simulink model "escooter_behavior_diagram"  (R2025b)
settings: Solver=VariableStepDiscrete  StartTime=0.0  StopTime=10.0  MaxStep=Inf  RelTol=1e-3
settings Model: Creator=320236370  LastModifiedBy=320236370

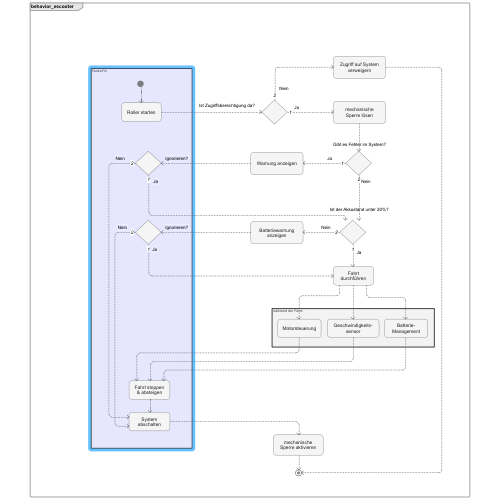
[thumbnail: Simulink's stored preview of the top-level diagram]
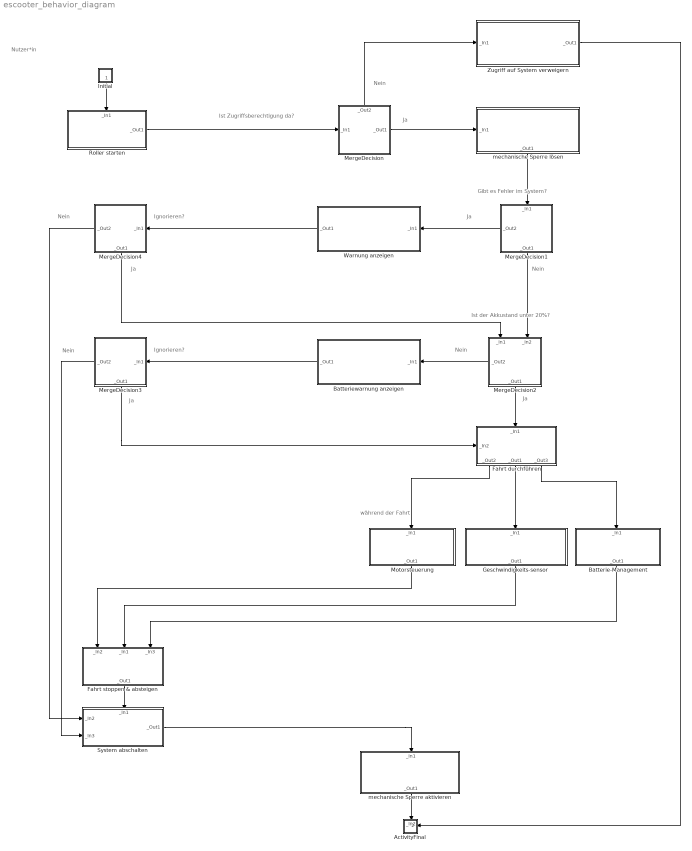
== system escooter_behavior_diagram ==
  note: Nein
  note: Nein
  note: Nein
  note: Ja
  note: Ignorieren?
  note: Ja
  note: Nutzer*in
  note: Nein
  note: Ja
  note: Ja
  note: während der Fahrt
  note: Nein
  note: Ist der Akkustand unter 20%?
  note: Gibt es Fehler im System?
  note: Ist Zugriffsberechtigung da?
  note: Ignorieren?
  note: Ja
  ActivityFinal : Subsystem
      settings: CopyFcn=set_param(gcbh,'LinkStatus','none');  PortSchema="{\"entries\":[{\"content\":{\"sides\":[{\"content\":{},\"type\":\"ConnectorPlacement.EquallySpacedRectSide\",\"uuid\":\"580456de-e9a6-4e12-b06b-ec681aee9b48\"},{\"content\":{\"connectorIds\":[\"In2\"],\"side\":\"RIGHT\"},\"type\":\"ConnectorPlacement.EquallySpacedRectSide\",\"uuid\":\"ad7fe46f-cc13-430b-9dbb-2068cc33ac37\"},{\"content\":{\"connectorIds\":[\"In1\"],\"side\":\"TOP\"},\"type\":\"ConnectorPlacement.EquallySpacedRectSide\",\"uuid\":\"5335bace-8b6a-45fe-956d-2b246f778999\"}]},\"type\":\"ConnectorPlacement.EquallySpacedConnector\",\"uuid\":\"e571f44c-7643-4dd6-8fcd-99f91b8b3e71\"}],\"packageUris\":[\"http://schema.mathworks.com/mf0/Connector/R2020b\"],\"version\":\"1.0\"}"
  Batterie-Management : Subsystem
      settings: CopyFcn=set_param(gcbh,'LinkStatus','none');  PortSchema="{\"entries\":[{\"content\":{\"sides\":[{\"content\":{},\"type\":\"ConnectorPlacement.EquallySpacedRectSide\",\"uuid\":\"580456de-e9a6-4e12-b06b-ec681aee9b48\"},{\"content\":{\"side\":\"RIGHT\"},\"type\":\"ConnectorPlacement.EquallySpacedRectSide\",\"uuid\":\"ad7fe46f-cc13-430b-9dbb-2068cc33ac37\"},{\"content\":{\"connectorIds\":[\"In1\"],\"side\":\"TOP\"},\"type\":\"ConnectorPlacement.EquallySpacedRectSide\",\"uuid\":\"5335bace-8b6a-45fe-956d-2b246f778999\"},{\"content\":{\"connectorIds\":[\"Out1\"],\"side\":\"BOTTOM\"},\"type\":\"ConnectorPlacement.EquallySpacedRectSide\",\"uuid\":\"4e917380-1660-449a-95a8-cd140500cc69\"}]},\"type\":\"ConnectorPlacement.EquallySpacedConnector\",\"uuid\":\"e571f44c-7643-4dd6-8fcd-99f91b8b3e71\"}],\"packageUris\":[\"http://schema.mathworks.com/mf0/Connector/R2020b\"],\"version\":\"1.0\"}"
  Batteriewarnung anzeigen : Subsystem
      settings: CopyFcn=set_param(gcbh,'LinkStatus','none');  PortSchema="{\"entries\":[{\"content\":{\"sides\":[{\"content\":{\"connectorIds\":[\"Out1\"]},\"type\":\"ConnectorPlacement.EquallySpacedRectSide\",\"uuid\":\"580456de-e9a6-4e12-b06b-ec681aee9b48\"},{\"content\":{\"connectorIds\":[\"In1\"],\"side\":\"RIGHT\"},\"type\":\"ConnectorPlacement.EquallySpacedRectSide\",\"uuid\":\"ad7fe46f-cc13-430b-9dbb-2068cc33ac37\"},{\"content\":{\"side\":\"TOP\"},\"type\":\"ConnectorPlacement.EquallySpacedRectSide\",\"uuid\":\"5335bace-8b6a-45fe-956d-2b246f778999\"},{\"content\":{\"side\":\"BOTTOM\"},\"type\":\"ConnectorPlacement.EquallySpacedRectSide\",\"uuid\":\"4e917380-1660-449a-95a8-cd140500cc69\"}]},\"type\":\"ConnectorPlacement.EquallySpacedConnector\",\"uuid\":\"e571f44c-7643-4dd6-8fcd-99f91b8b3e71\"}],\"packageUris\":[\"http://schema.mathworks.com/mf0/Connector/R2020b\"],\"version\":\"1.0\"}"
  Fahrt durchführen : Subsystem
      settings: CopyFcn=set_param(gcbh,'LinkStatus','none');  PortSchema="{\"entries\":[{\"content\":{\"sides\":[{\"content\":{\"connectorIds\":[\"In1\"]},\"type\":\"ConnectorPlacement.EquallySpacedRectSide\",\"uuid\":\"580456de-e9a6-4e12-b06b-ec681aee9b48\"},{\"content\":{\"side\":\"RIGHT\"},\"type\":\"ConnectorPlacement.EquallySpacedRectSide\",\"uuid\":\"ad7fe46f-cc13-430b-9dbb-2068cc33ac37\"},{\"content\":{\"connectorIds\":[\"In2\"],\"side\":\"TOP\"},\"type\":\"ConnectorPlacement.EquallySpacedRectSide\",\"uuid\":\"5335bace-8b6a-45fe-956d-2b246f778999\"},{\"content\":{\"connectorIds\":[\"Out1\",\"Out2\",\"Out3\"],\"side\":\"BOTTOM\"},\"type\":\"ConnectorPlacement.EquallySpacedRectSide\",\"uuid\":\"4e917380-1660-449a-95a8-cd140500cc69\"}]},\"type\":\"ConnectorPlacement.EquallySpacedConnector\",\"uuid\":\"e571f44c-7643-4dd6-8fcd-99f91b8b3e71\"}],\"packageUris\":[\"http://schema.mathworks.com/mf0/Connector/R2020b\"],\"version\":\"1.0\"}"
  Fahrt stoppen & absteigen : Subsystem
      settings: CopyFcn=set_param(gcbh,'LinkStatus','none');  PortSchema="{\"entries\":[{\"content\":{\"sides\":[{\"content\":{},\"type\":\"ConnectorPlacement.EquallySpacedRectSide\",\"uuid\":\"580456de-e9a6-4e12-b06b-ec681aee9b48\"},{\"content\":{\"side\":\"RIGHT\"},\"type\":\"ConnectorPlacement.EquallySpacedRectSide\",\"uuid\":\"ad7fe46f-cc13-430b-9dbb-2068cc33ac37\"},{\"content\":{\"connectorIds\":[\"In1\",\"In2\",\"In3\"],\"side\":\"TOP\"},\"type\":\"ConnectorPlacement.EquallySpacedRectSide\",\"uuid\":\"5335bace-8b6a-45fe-956d-2b246f778999\"},{\"content\":{\"connectorIds\":[\"Out1\"],\"side\":\"BOTTOM\"},\"type\":\"ConnectorPlacement.EquallySpacedRectSide\",\"uuid\":\"4e917380-1660-449a-95a8-cd140500cc69\"}]},\"type\":\"ConnectorPlacement.EquallySpacedConnector\",\"uuid\":\"e571f44c-7643-4dd6-8fcd-99f91b8b3e71\"}],\"packageUris\":[\"http://schema.mathworks.com/mf0/Connector/R2020b\"],\"version\":\"1.0\"}"
  Geschwindigkeits-sensor : Subsystem
      settings: CopyFcn=set_param(gcbh,'LinkStatus','none');  PortSchema="{\"entries\":[{\"content\":{\"sides\":[{\"content\":{},\"type\":\"ConnectorPlacement.EquallySpacedRectSide\",\"uuid\":\"580456de-e9a6-4e12-b06b-ec681aee9b48\"},{\"content\":{\"side\":\"RIGHT\"},\"type\":\"ConnectorPlacement.EquallySpacedRectSide\",\"uuid\":\"ad7fe46f-cc13-430b-9dbb-2068cc33ac37\"},{\"content\":{\"connectorIds\":[\"In1\"],\"side\":\"TOP\"},\"type\":\"ConnectorPlacement.EquallySpacedRectSide\",\"uuid\":\"5335bace-8b6a-45fe-956d-2b246f778999\"},{\"content\":{\"connectorIds\":[\"Out1\"],\"side\":\"BOTTOM\"},\"type\":\"ConnectorPlacement.EquallySpacedRectSide\",\"uuid\":\"4e917380-1660-449a-95a8-cd140500cc69\"}]},\"type\":\"ConnectorPlacement.EquallySpacedConnector\",\"uuid\":\"e571f44c-7643-4dd6-8fcd-99f91b8b3e71\"}],\"packageUris\":[\"http://schema.mathworks.com/mf0/Connector/R2020b\"],\"version\":\"1.0\"}"
  Initial : Subsystem
      settings: CopyFcn=set_param(gcbh,'LinkStatus','none');  PortSchema="{\"entries\":[{\"content\":{\"sides\":[{\"content\":{},\"type\":\"ConnectorPlacement.EquallySpacedRectSide\",\"uuid\":\"580456de-e9a6-4e12-b06b-ec681aee9b48\"},{\"content\":{\"side\":\"RIGHT\"},\"type\":\"ConnectorPlacement.EquallySpacedRectSide\",\"uuid\":\"ad7fe46f-cc13-430b-9dbb-2068cc33ac37\"},{\"content\":{\"side\":\"TOP\"},\"type\":\"ConnectorPlacement.EquallySpacedRectSide\",\"uuid\":\"5335bace-8b6a-45fe-956d-2b246f778999\"},{\"content\":{\"connectorIds\":[\"Out1\"],\"side\":\"BOTTOM\"},\"type\":\"ConnectorPlacement.EquallySpacedRectSide\",\"uuid\":\"ed4f2dcd-de42-45b1-90c6-13ee85adcd8c\"}]},\"type\":\"ConnectorPlacement.EquallySpacedConnector\",\"uuid\":\"e571f44c-7643-4dd6-8fcd-99f91b8b3e71\"}],\"packageUris\":[\"http://schema.mathworks.com/mf0/Connector/R2020b\"],\"version\":\"1.0\"}"
  MergeDecision : Subsystem
      settings: CopyFcn=set_param(gcbh,'LinkStatus','none');  PortSchema="{\"entries\":[{\"content\":{\"sides\":[{\"content\":{\"connectorIds\":[\"In1\"]},\"type\":\"ConnectorPlacement.EquallySpacedRectSide\",\"uuid\":\"580456de-e9a6-4e12-b06b-ec681aee9b48\"},{\"content\":{\"connectorIds\":[\"Out2\"],\"side\":\"RIGHT\"},\"type\":\"ConnectorPlacement.EquallySpacedRectSide\",\"uuid\":\"ad7fe46f-cc13-430b-9dbb-2068cc33ac37\"},{\"content\":{\"connectorIds\":[\"Out1\"],\"side\":\"TOP\"},\"type\":\"ConnectorPlacement.EquallySpacedRectSide\",\"uuid\":\"5335bace-8b6a-45fe-956d-2b246f778999\"}]},\"type\":\"ConnectorPlacement.EquallySpacedConnector\",\"uuid\":\"e571f44c-7643-4dd6-8fcd-99f91b8b3e71\"}],\"packageUris\":[\"http://schema.mathworks.com/mf0/Connector/R2020b\"],\"version\":\"1.0\"}"
  MergeDecision1 : Subsystem
      settings: CopyFcn=set_param(gcbh,'LinkStatus','none');  PortSchema="{\"entries\":[{\"content\":{\"sides\":[{\"content\":{\"connectorIds\":[\"Out2\"]},\"type\":\"ConnectorPlacement.EquallySpacedRectSide\",\"uuid\":\"580456de-e9a6-4e12-b06b-ec681aee9b48\"},{\"content\":{\"side\":\"RIGHT\"},\"type\":\"ConnectorPlacement.EquallySpacedRectSide\",\"uuid\":\"ad7fe46f-cc13-430b-9dbb-2068cc33ac37\"},{\"content\":{\"connectorIds\":[\"In1\"],\"side\":\"TOP\"},\"type\":\"ConnectorPlacement.EquallySpacedRectSide\",\"uuid\":\"5335bace-8b6a-45fe-956d-2b246f778999\"},{\"content\":{\"connectorIds\":[\"Out1\"],\"side\":\"BOTTOM\"},\"type\":\"ConnectorPlacement.EquallySpacedRectSide\",\"uuid\":\"6c820d2e-b5ae-4678-8c2b-f20977a1622f\"}]},\"type\":\"ConnectorPlacement.EquallySpacedConnector\",\"uuid\":\"e571f44c-7643-4dd6-8fcd-99f91b8b3e71\"}],\"packageUris\":[\"http://schema.mathworks.com/mf0/Connector/R2020b\"],\"version\":\"1.0\"}"
  MergeDecision2 : Subsystem
      settings: CopyFcn=set_param(gcbh,'LinkStatus','none');  PortSchema="{\"entries\":[{\"content\":{\"sides\":[{\"content\":{\"connectorIds\":[\"Out1\"]},\"type\":\"ConnectorPlacement.EquallySpacedRectSide\",\"uuid\":\"580456de-e9a6-4e12-b06b-ec681aee9b48\"},{\"content\":{\"side\":\"RIGHT\"},\"type\":\"ConnectorPlacement.EquallySpacedRectSide\",\"uuid\":\"ad7fe46f-cc13-430b-9dbb-2068cc33ac37\"},{\"content\":{\"connectorIds\":[\"In1\",\"In2\"],\"side\":\"TOP\"},\"type\":\"ConnectorPlacement.EquallySpacedRectSide\",\"uuid\":\"5335bace-8b6a-45fe-956d-2b246f778999\"},{\"content\":{\"connectorIds\":[\"Out2\"],\"side\":\"BOTTOM\"},\"type\":\"ConnectorPlacement.EquallySpacedRectSide\",\"uuid\":\"8081780a-9cab-4486-9f8d-54582980b840\"}]},\"type\":\"ConnectorPlacement.EquallySpacedConnector\",\"uuid\":\"e571f44c-7643-4dd6-8fcd-99f91b8b3e71\"}],\"packageUris\":[\"http://schema.mathworks.com/mf0/Connector/R2020b\"],\"version\":\"1.0\"}"
  MergeDecision3 : Subsystem
      settings: CopyFcn=set_param(gcbh,'LinkStatus','none');  PortSchema="{\"entries\":[{\"content\":{\"sides\":[{\"content\":{\"connectorIds\":[\"Out1\"]},\"type\":\"ConnectorPlacement.EquallySpacedRectSide\",\"uuid\":\"580456de-e9a6-4e12-b06b-ec681aee9b48\"},{\"content\":{\"connectorIds\":[\"In1\"],\"side\":\"RIGHT\"},\"type\":\"ConnectorPlacement.EquallySpacedRectSide\",\"uuid\":\"ad7fe46f-cc13-430b-9dbb-2068cc33ac37\"},{\"content\":{\"side\":\"TOP\"},\"type\":\"ConnectorPlacement.EquallySpacedRectSide\",\"uuid\":\"5335bace-8b6a-45fe-956d-2b246f778999\"},{\"content\":{\"connectorIds\":[\"Out2\"],\"side\":\"BOTTOM\"},\"type\":\"ConnectorPlacement.EquallySpacedRectSide\",\"uuid\":\"8081780a-9cab-4486-9f8d-54582980b840\"}]},\"type\":\"ConnectorPlacement.EquallySpacedConnector\",\"uuid\":\"e571f44c-7643-4dd6-8fcd-99f91b8b3e71\"}],\"packageUris\":[\"http://schema.mathworks.com/mf0/Connector/R2020b\"],\"version\":\"1.0\"}"
  MergeDecision4 : Subsystem
      settings: CopyFcn=set_param(gcbh,'LinkStatus','none');  PortSchema="{\"entries\":[{\"content\":{\"sides\":[{\"content\":{\"connectorIds\":[\"Out1\"]},\"type\":\"ConnectorPlacement.EquallySpacedRectSide\",\"uuid\":\"580456de-e9a6-4e12-b06b-ec681aee9b48\"},{\"content\":{\"connectorIds\":[\"In1\"],\"side\":\"RIGHT\"},\"type\":\"ConnectorPlacement.EquallySpacedRectSide\",\"uuid\":\"ad7fe46f-cc13-430b-9dbb-2068cc33ac37\"},{\"content\":{\"side\":\"TOP\"},\"type\":\"ConnectorPlacement.EquallySpacedRectSide\",\"uuid\":\"5335bace-8b6a-45fe-956d-2b246f778999\"},{\"content\":{\"connectorIds\":[\"Out2\"],\"side\":\"BOTTOM\"},\"type\":\"ConnectorPlacement.EquallySpacedRectSide\",\"uuid\":\"8081780a-9cab-4486-9f8d-54582980b840\"}]},\"type\":\"ConnectorPlacement.EquallySpacedConnector\",\"uuid\":\"e571f44c-7643-4dd6-8fcd-99f91b8b3e71\"}],\"packageUris\":[\"http://schema.mathworks.com/mf0/Connector/R2020b\"],\"version\":\"1.0\"}"
  Motorsteuerung : Subsystem
      settings: CopyFcn=set_param(gcbh,'LinkStatus','none');  PortSchema="{\"entries\":[{\"content\":{\"sides\":[{\"content\":{},\"type\":\"ConnectorPlacement.EquallySpacedRectSide\",\"uuid\":\"580456de-e9a6-4e12-b06b-ec681aee9b48\"},{\"content\":{\"side\":\"RIGHT\"},\"type\":\"ConnectorPlacement.EquallySpacedRectSide\",\"uuid\":\"ad7fe46f-cc13-430b-9dbb-2068cc33ac37\"},{\"content\":{\"connectorIds\":[\"In1\"],\"side\":\"TOP\"},\"type\":\"ConnectorPlacement.EquallySpacedRectSide\",\"uuid\":\"5335bace-8b6a-45fe-956d-2b246f778999\"},{\"content\":{\"connectorIds\":[\"Out1\"],\"side\":\"BOTTOM\"},\"type\":\"ConnectorPlacement.EquallySpacedRectSide\",\"uuid\":\"4e917380-1660-449a-95a8-cd140500cc69\"}]},\"type\":\"ConnectorPlacement.EquallySpacedConnector\",\"uuid\":\"e571f44c-7643-4dd6-8fcd-99f91b8b3e71\"}],\"packageUris\":[\"http://schema.mathworks.com/mf0/Connector/R2020b\"],\"version\":\"1.0\"}"
  Roller starten : Subsystem
      settings: CopyFcn=set_param(gcbh,'LinkStatus','none');  PortSchema="{\"entries\":[{\"content\":{\"sides\":[{\"content\":{},\"type\":\"ConnectorPlacement.EquallySpacedRectSide\",\"uuid\":\"580456de-e9a6-4e12-b06b-ec681aee9b48\"},{\"content\":{\"connectorIds\":[\"Out1\"],\"side\":\"RIGHT\"},\"type\":\"ConnectorPlacement.EquallySpacedRectSide\",\"uuid\":\"ad7fe46f-cc13-430b-9dbb-2068cc33ac37\"},{\"content\":{\"connectorIds\":[\"In1\"],\"side\":\"TOP\"},\"type\":\"ConnectorPlacement.EquallySpacedRectSide\",\"uuid\":\"5335bace-8b6a-45fe-956d-2b246f778999\"},{\"content\":{\"side\":\"BOTTOM\"},\"type\":\"ConnectorPlacement.EquallySpacedRectSide\",\"uuid\":\"4e917380-1660-449a-95a8-cd140500cc69\"}]},\"type\":\"ConnectorPlacement.EquallySpacedConnector\",\"uuid\":\"e571f44c-7643-4dd6-8fcd-99f91b8b3e71\"}],\"packageUris\":[\"http://schema.mathworks.com/mf0/Connector/R2020b\"],\"version\":\"1.0\"}"
  System abschalten : Subsystem
      settings: CopyFcn=set_param(gcbh,'LinkStatus','none');  PortSchema="{\"entries\":[{\"content\":{\"sides\":[{\"content\":{\"connectorIds\":[\"In2\",\"In3\"]},\"type\":\"ConnectorPlacement.EquallySpacedRectSide\",\"uuid\":\"580456de-e9a6-4e12-b06b-ec681aee9b48\"},{\"content\":{\"connectorIds\":[\"Out1\"],\"side\":\"RIGHT\"},\"type\":\"ConnectorPlacement.EquallySpacedRectSide\",\"uuid\":\"ad7fe46f-cc13-430b-9dbb-2068cc33ac37\"},{\"content\":{\"connectorIds\":[\"In1\"],\"side\":\"TOP\"},\"type\":\"ConnectorPlacement.EquallySpacedRectSide\",\"uuid\":\"5335bace-8b6a-45fe-956d-2b246f778999\"},{\"content\":{\"side\":\"BOTTOM\"},\"type\":\"ConnectorPlacement.EquallySpacedRectSide\",\"uuid\":\"4e917380-1660-449a-95a8-cd140500cc69\"}]},\"type\":\"ConnectorPlacement.EquallySpacedConnector\",\"uuid\":\"e571f44c-7643-4dd6-8fcd-99f91b8b3e71\"}],\"packageUris\":[\"http://schema.mathworks.com/mf0/Connector/R2020b\"],\"version\":\"1.0\"}"
  Warnung anzeigen : Subsystem
      settings: CopyFcn=set_param(gcbh,'LinkStatus','none');  PortSchema="{\"entries\":[{\"content\":{\"sides\":[{\"content\":{\"connectorIds\":[\"Out1\"]},\"type\":\"ConnectorPlacement.EquallySpacedRectSide\",\"uuid\":\"580456de-e9a6-4e12-b06b-ec681aee9b48\"},{\"content\":{\"connectorIds\":[\"In1\"],\"side\":\"RIGHT\"},\"type\":\"ConnectorPlacement.EquallySpacedRectSide\",\"uuid\":\"ad7fe46f-cc13-430b-9dbb-2068cc33ac37\"},{\"content\":{\"side\":\"TOP\"},\"type\":\"ConnectorPlacement.EquallySpacedRectSide\",\"uuid\":\"5335bace-8b6a-45fe-956d-2b246f778999\"},{\"content\":{\"side\":\"BOTTOM\"},\"type\":\"ConnectorPlacement.EquallySpacedRectSide\",\"uuid\":\"4e917380-1660-449a-95a8-cd140500cc69\"}]},\"type\":\"ConnectorPlacement.EquallySpacedConnector\",\"uuid\":\"e571f44c-7643-4dd6-8fcd-99f91b8b3e71\"}],\"packageUris\":[\"http://schema.mathworks.com/mf0/Connector/R2020b\"],\"version\":\"1.0\"}"
  Zugriff auf System verweigern : Subsystem
      settings: CopyFcn=set_param(gcbh,'LinkStatus','none');  PortSchema="{\"entries\":[{\"content\":{\"sides\":[{\"content\":{\"connectorIds\":[\"In1\"]},\"type\":\"ConnectorPlacement.EquallySpacedRectSide\",\"uuid\":\"580456de-e9a6-4e12-b06b-ec681aee9b48\"},{\"content\":{\"connectorIds\":[\"Out1\"],\"side\":\"RIGHT\"},\"type\":\"ConnectorPlacement.EquallySpacedRectSide\",\"uuid\":\"ad7fe46f-cc13-430b-9dbb-2068cc33ac37\"},{\"content\":{\"side\":\"TOP\"},\"type\":\"ConnectorPlacement.EquallySpacedRectSide\",\"uuid\":\"5335bace-8b6a-45fe-956d-2b246f778999\"},{\"content\":{\"side\":\"BOTTOM\"},\"type\":\"ConnectorPlacement.EquallySpacedRectSide\",\"uuid\":\"4e917380-1660-449a-95a8-cd140500cc69\"}]},\"type\":\"ConnectorPlacement.EquallySpacedConnector\",\"uuid\":\"e571f44c-7643-4dd6-8fcd-99f91b8b3e71\"}],\"packageUris\":[\"http://schema.mathworks.com/mf0/Connector/R2020b\"],\"version\":\"1.0\"}"
  mechanische Sperre aktivieren : Subsystem
      settings: CopyFcn=set_param(gcbh,'LinkStatus','none');  PortSchema="{\"entries\":[{\"content\":{\"sides\":[{\"content\":{},\"type\":\"ConnectorPlacement.EquallySpacedRectSide\",\"uuid\":\"580456de-e9a6-4e12-b06b-ec681aee9b48\"},{\"content\":{\"side\":\"RIGHT\"},\"type\":\"ConnectorPlacement.EquallySpacedRectSide\",\"uuid\":\"ad7fe46f-cc13-430b-9dbb-2068cc33ac37\"},{\"content\":{\"connectorIds\":[\"In1\"],\"side\":\"TOP\"},\"type\":\"ConnectorPlacement.EquallySpacedRectSide\",\"uuid\":\"5335bace-8b6a-45fe-956d-2b246f778999\"},{\"content\":{\"connectorIds\":[\"Out1\"],\"side\":\"BOTTOM\"},\"type\":\"ConnectorPlacement.EquallySpacedRectSide\",\"uuid\":\"4e917380-1660-449a-95a8-cd140500cc69\"}]},\"type\":\"ConnectorPlacement.EquallySpacedConnector\",\"uuid\":\"e571f44c-7643-4dd6-8fcd-99f91b8b3e71\"}],\"packageUris\":[\"http://schema.mathworks.com/mf0/Connector/R2020b\"],\"version\":\"1.0\"}"
  mechanische Sperre lösen : Subsystem
      settings: CopyFcn=set_param(gcbh,'LinkStatus','none');  PortSchema="{\"entries\":[{\"content\":{\"sides\":[{\"content\":{\"connectorIds\":[\"In1\"]},\"type\":\"ConnectorPlacement.EquallySpacedRectSide\",\"uuid\":\"580456de-e9a6-4e12-b06b-ec681aee9b48\"},{\"content\":{\"side\":\"RIGHT\"},\"type\":\"ConnectorPlacement.EquallySpacedRectSide\",\"uuid\":\"ad7fe46f-cc13-430b-9dbb-2068cc33ac37\"},{\"content\":{\"side\":\"TOP\"},\"type\":\"ConnectorPlacement.EquallySpacedRectSide\",\"uuid\":\"5335bace-8b6a-45fe-956d-2b246f778999\"},{\"content\":{\"connectorIds\":[\"Out1\"],\"side\":\"BOTTOM\"},\"type\":\"ConnectorPlacement.EquallySpacedRectSide\",\"uuid\":\"4e917380-1660-449a-95a8-cd140500cc69\"}]},\"type\":\"ConnectorPlacement.EquallySpacedConnector\",\"uuid\":\"e571f44c-7643-4dd6-8fcd-99f91b8b3e71\"}],\"packageUris\":[\"http://schema.mathworks.com/mf0/Connector/R2020b\"],\"version\":\"1.0\"}"
  wires:
  MergeDecision/2(_Out1) -> mechanische Sperre lösen/1(_In1)
  mechanische Sperre lösen/1(_Out1) -> MergeDecision1/1(_In1)
  MergeDecision2/2(_Out1) -> Fahrt durchführen/2(_In1)
  Fahrt durchführen/2(_Out1) -> Geschwindigkeits-sensor/1(_In1)
  Fahrt durchführen/1(_Out2) -> Motorsteuerung/1(_In1)
  Fahrt durchführen/3(_Out3) -> Batterie-Management/1(_In1)
  MergeDecision1/2(_Out2) -> Warnung anzeigen/1(_In1)
  MergeDecision2/1(_Out2) -> Batteriewarnung anzeigen/1(_In1)
  Roller starten/1(_Out1) -> MergeDecision/1(_In1)
  Initial/1(_Out1) -> Roller starten/1(_In1)
  Batteriewarnung anzeigen/1(_Out1) -> MergeDecision3/1(_In1)
  MergeDecision3/2(_Out1) -> Fahrt durchführen/1(_In2)
  Warnung anzeigen/1(_Out1) -> MergeDecision4/1(_In1)
  MergeDecision4/2(_Out1) -> MergeDecision2/1(_In1)
  MergeDecision1/1(_Out1) -> MergeDecision2/2(_In2)
  MergeDecision/1(_Out2) -> Zugriff auf System verweigern/1(_In1)
  Zugriff auf System verweigern/1(_Out1) -> ActivityFinal/2(_In1)
  Geschwindigkeits-sensor/1(_Out1) -> Fahrt stoppen & absteigen/2(_In1)
  Motorsteuerung/1(_Out1) -> Fahrt stoppen & absteigen/1(_In2)
  Batterie-Management/1(_Out1) -> Fahrt stoppen & absteigen/3(_In3)
  MergeDecision4/1(_Out2) -> System abschalten/2(_In2)
  MergeDecision3/1(_Out2) -> System abschalten/3(_In3)
  mechanische Sperre aktivieren/1(_Out1) -> ActivityFinal/1(_In2)
  Fahrt stoppen & absteigen/1(_Out1) -> System abschalten/1(_In1)
  System abschalten/1(_Out1) -> mechanische Sperre aktivieren/1(_In1)

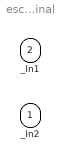
== system escooter_behavior_diagram/ActivityFinal ==
  _In2 : Inport
  _In1 : Inport  Port=2

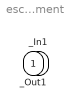
== system escooter_behavior_diagram/Batterie-Management ==
  _In1 : Inport
  _Out1 : Outport

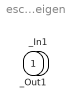
== system escooter_behavior_diagram/Batteriewarnung anzeigen ==
  _In1 : Inport
  _Out1 : Outport

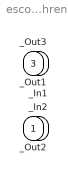
== system escooter_behavior_diagram/Fahrt durchführen ==
  _In2 : Inport
  _In1 : Inport  Port=2
  _Out2 : Outport
  _Out1 : Outport  Port=2
  _Out3 : Outport  Port=3

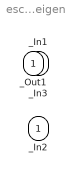
== system escooter_behavior_diagram/Fahrt stoppen & absteigen ==
  _In2 : Inport
  _In1 : Inport  Port=2
  _In3 : Inport  Port=3
  _Out1 : Outport

== system escooter_behavior_diagram/Geschwindigkeits-sensor ==
  _In1 : Inport
  _Out1 : Outport

== system escooter_behavior_diagram/Initial ==
  _Out1 : Outport

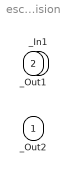
== system escooter_behavior_diagram/MergeDecision ==
  _In1 : Inport
  _Out2 : Outport
  _Out1 : Outport  Port=2

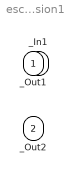
== system escooter_behavior_diagram/MergeDecision1 ==
  _In1 : Inport
  _Out1 : Outport
  _Out2 : Outport  Port=2

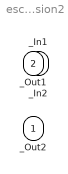
== system escooter_behavior_diagram/MergeDecision2 ==
  _In1 : Inport
  _In2 : Inport  Port=2
  _Out2 : Outport
  _Out1 : Outport  Port=2

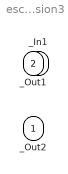
== system escooter_behavior_diagram/MergeDecision3 ==
  _In1 : Inport
  _Out2 : Outport
  _Out1 : Outport  Port=2

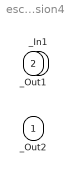
== system escooter_behavior_diagram/MergeDecision4 ==
  _In1 : Inport
  _Out2 : Outport
  _Out1 : Outport  Port=2

== system escooter_behavior_diagram/Motorsteuerung ==
  _In1 : Inport
  _Out1 : Outport

== system escooter_behavior_diagram/Roller starten ==
  _In1 : Inport
  _Out1 : Outport

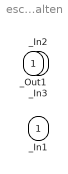
== system escooter_behavior_diagram/System abschalten ==
  _In1 : Inport
  _In2 : Inport  Port=2
  _In3 : Inport  Port=3
  _Out1 : Outport

== system escooter_behavior_diagram/Warnung anzeigen ==
  _In1 : Inport
  _Out1 : Outport

== system escooter_behavior_diagram/Zugriff auf System verweigern ==
  _In1 : Inport
  _Out1 : Outport

== system escooter_behavior_diagram/mechanische Sperre aktivieren ==
  _In1 : Inport
  _Out1 : Outport

== system escooter_behavior_diagram/mechanische Sperre lösen ==
  _In1 : Inport
  _Out1 : Outport
